simulink model "ADHW6p4"  (R2022b)
settings: Solver=VariableStepAuto  StartTime=0.0  StopTime=1800.0  RelTol=1e-3
settings Model: Creator=izacu  LastModifiedBy=izacu

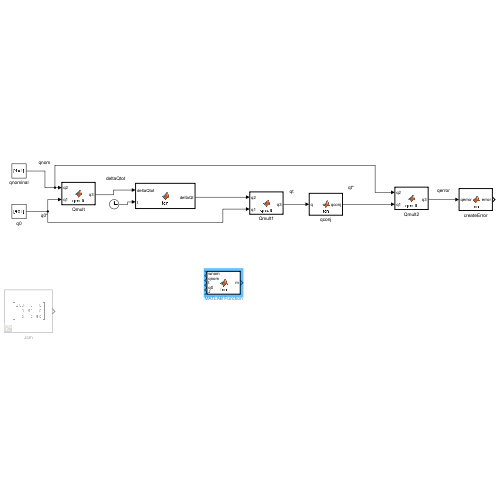
[thumbnail: Simulink's stored preview of the top-level diagram]
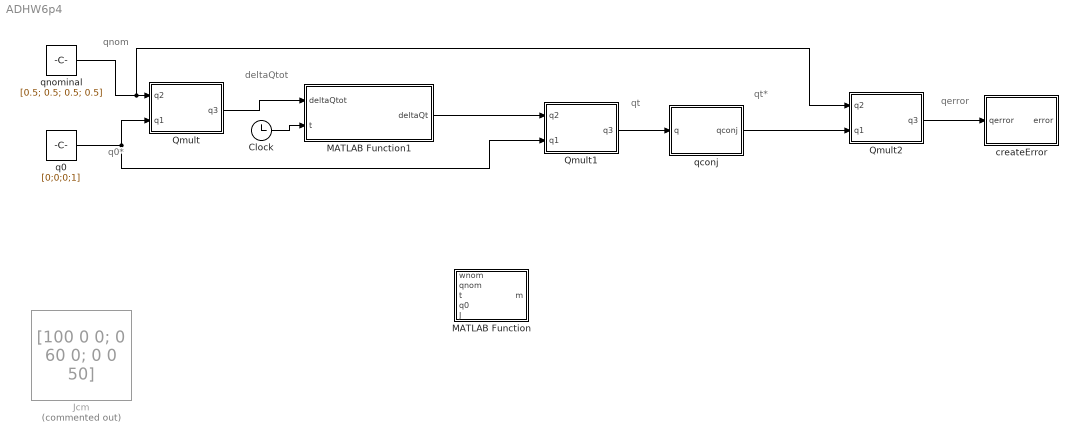
== system ADHW6p4 ==
  note: qerror
  note: qt*
  note: qt
  note: qnom
  note: q0*
  note: deltaQtot
  Clock : Clock
  Jcm : Constant  Commented=on  Value=[100 0 0; 0 60 0; 0 0 50]
  MATLAB Function : MATLAB Function  TreatAsAtomicUnit=on
  MATLAB Function1 : MATLAB Function  TreatAsAtomicUnit=on
  Qmult : MATLAB Function  TreatAsAtomicUnit=on
  Qmult1 : MATLAB Function  TreatAsAtomicUnit=on
  Qmult2 : MATLAB Function  TreatAsAtomicUnit=on
  createError : MATLAB Function  TreatAsAtomicUnit=on
  q0 : Constant  Value=[0;0;0;1]
  qconj : MATLAB Function  TreatAsAtomicUnit=on
  qnominal : Constant  Value=[0.5; 0.5; 0.5; 0.5]
  wires:
  qnominal/1 -> Qmult2/1(q2), Qmult/1(q2)
  q0/1 -> Qmult1/2(q1), Qmult/2(q1)
  Qmult/1(q3) -> MATLAB Function1/1(deltaQtot)
  Clock/1 -> MATLAB Function1/2(t)
  MATLAB Function1/1(deltaQt) -> Qmult1/1(q2)
  Qmult1/1(q3) -> qconj/1(q)
  qconj/1(qconj) -> Qmult2/2(q1)
  Qmult2/1(q3) -> createError/1(qerror)

== matlab function ADHW6p4/MATLAB Function1 ==
  data: deltaQtot input; deltaQt output; t input
function deltaQt = fcn(deltaQtot,t)

t1 = 1800;

deltaThetatot = 2*acos(deltaQtot(4));

deltaThetat = (deltaThetatot/t1) * (t);

e = deltaQtot(1:3)./sin(deltaThetatot/2);

deltaQt = zeros(4,1);

deltaQt(4) = cos(deltaThetat/2);

deltaQt(1:3) = sin(deltaThetat/2).*e;

== matlab function ADHW6p4/Qmult1 ==
  data: q2 input; q1 input; q3 output
function q3 = qmult(q2,q1)

q3 = [q2(4).*q1(1:3) + q1(4).*q2(1:3) - cross(q2(1:3),q1(1:3));
    q2(4)*q1(4) - dot(q2(1:3),q1(1:3))];

== matlab function ADHW6p4/qconj ==
  data: q input; qconj output
function qconj = fcn(q)
qconj = q;
qconj(1:3) = -q(1:3);

== matlab function ADHW6p4/Qmult ==
  data: q2 input; q1 input; q3 output
function q3 = qmult(q2,q1)

q3 = [q2(4).*q1(1:3) + q1(4).*q2(1:3) - cross(q2(1:3),q1(1:3));
    q2(4)*q1(4) - dot(q2(1:3),q1(1:3))];

== matlab function ADHW6p4/Qmult2 ==
  data: q2 input; q1 input; q3 output
function q3 = qmult(q2,q1)

q3 = [q2(4).*q1(1:3) + q1(4).*q2(1:3) - cross(q2(1:3),q1(1:3));
    q2(4)*q1(4) - dot(q2(1:3),q1(1:3))];

== matlab function ADHW6p4/createError ==
  data: qerror input; error output
function error = fcn(qerror)

error = 2*qerror(1:3);

error = error / qerror(4);

== matlab function ADHW6p4/MATLAB Function ==
  data: wnom input; m output; qnom input; t input; q0 input; J input
function m = fcn(wnom,qnom,t,q0,J)

deltaQ = 0;
y = u;
